simulink model "4ex4_sim"  (R2015b)
settings: Solver=VariableStepAuto  StartTime=0.0  StopTime=5  RelTol=1e-3
values from neighbouring files (symbols this model uses):
  J = (J1 + J2)    (= 3.6e-05)    [ex1.m]    (also in ex2.m; ex3.m; ex4.m)
  motor_L = motor_pars    [ex1.m]    (also in ex2.m; ex3.m; ex4.m)
  n = 5    [ex1.m]    (also in ex2.m; ex3.m; ex4.m; ex5.m)
  sim_zoh_sample_time = 0    [ex2.m]    (also in ex3.m; ex4.m = 0.001; exall.m)
libraries: simulink x1
settings Model: Creator=gabras  LastModifiedBy=Lamn
settings SolverCC: ZeroCrossAlgorithm=Adaptive
settings DataIOCC: SaveFormat=Array
settings DebuggingCC: SolverPrmCheckMsg=warning
settings HardwareCC: ProdBitPerPointer=32  ProdLargestAtomicFloat=None  ProdIntDivRoundTo=Undefined  ProdEndianess=Unspecified  ProdWordSize=32  ProdHWDeviceType=32-bit Generic
settings GRTTargetCC: GeneratePreprocessorConditionals=Disable all
settings ConfigComp: CovModelRefEnable=Off  CovSFcnEnable=off

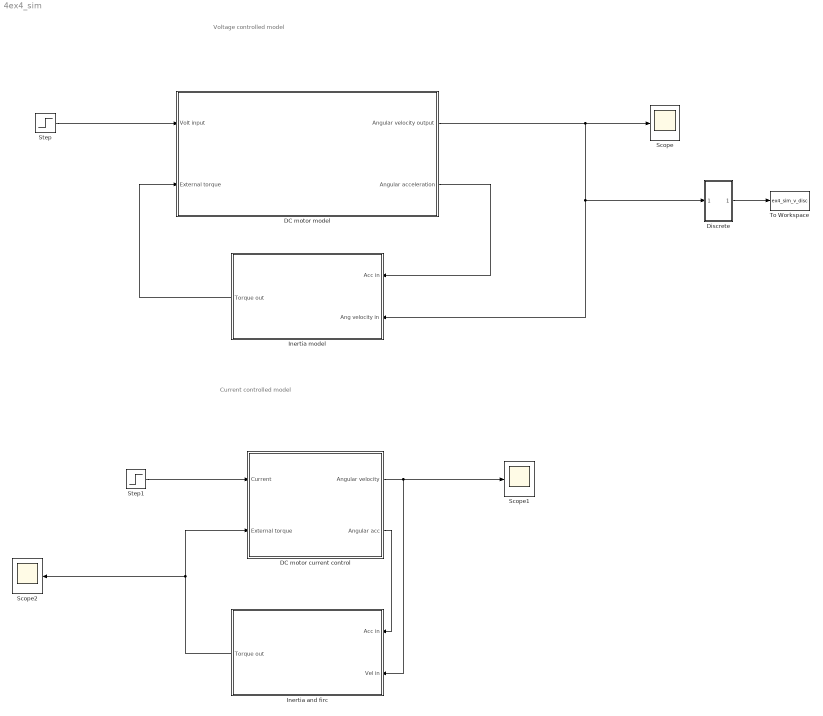
== system 4ex4_sim ==
  note: Current controlled model
  note: Voltage controlled model
  "DC motor current control " : Subsystem
  DC motor model : Subsystem
  Discrete : Subsystem
  Inertia and firc : Subsystem
  Inertia model : Subsystem
  Scope : Scope
  Scope1 : Scope
  Scope2 : Scope
  Step : Step  Time=0  SampleTime=0
  Step1 : Step  Time=0  SampleTime=0
  To Workspace : ToWorkspace  VariableName=ex4_sim_v_disc  SaveFormat=Timeseries  SampleTime=-1
  wires:
  Step/1 -> DC motor model/1("Volt input ")
  DC motor model/1("Angular velocity output ") -> Discrete/1(In1), Inertia model/2(Ang velocity in), Scope/1
  Inertia model/1(Torque out) -> DC motor model/2(External torque)
  DC motor model/2("Angular acceleration ") -> Inertia model/1(Acc in)
  Step1/1 -> "DC motor current control "/1(Current)
  "DC motor current control "/1(Angular velocity) -> Scope1/1, Inertia and firc/2(Vel in)
  "DC motor current control "/2(Angular acc) -> Inertia and firc/1(Acc in)
  Inertia and firc/1(Torque out) -> Scope2/1, "DC motor current control "/2(External torque)
  Discrete/1(Out1) -> To Workspace/1

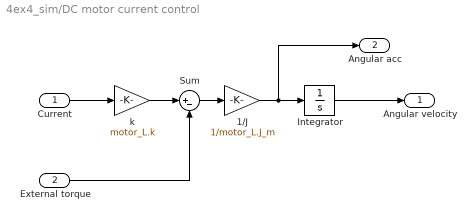
== system 4ex4_sim/DC motor current control  ==
  Current : Inport
  External torque : Inport  Port=2
  1/J : Gain  Gain=1/motor_L.J_m
  Integrator : Integrator
  Sum : Sum  Inputs=|+-
  "k " : Gain  Gain=motor_L.k
  Angular velocity : Outport
  Angular acc : Outport  Port=2
  wires:
  Current/1 -> "k "/1
  External torque/1 -> Sum/2
  "k "/1 -> Sum/1
  Sum/1 -> 1/J/1
  1/J/1 -> Angular acc/1, Integrator/1
  Integrator/1 -> Angular velocity/1

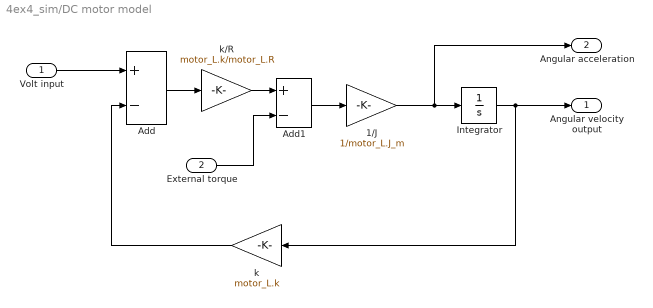
== system 4ex4_sim/DC motor model ==
  "Volt input " : Inport
  External torque : Inport  Port=2
  1/J : Gain  Gain=1/motor_L.J_m
  Add : Sum  Inputs=+-
  Add1 : Sum  Inputs=+-
  Integrator : Integrator
  k : Gain  Gain=motor_L.k
  "k/R " : Gain  Gain=motor_L.k/motor_L.R
  "Angular velocity output " : Outport
  "Angular acceleration " : Outport  Port=2
  wires:
  "Volt input "/1 -> Add/1
  k/1 -> Add/2
  Add/1 -> "k/R "/1
  "k/R "/1 -> Add1/1
  Add1/1 -> 1/J/1
  1/J/1 -> "Angular acceleration "/1, Integrator/1
  Integrator/1 -> k/1, "Angular velocity output "/1
  External torque/1 -> Add1/2

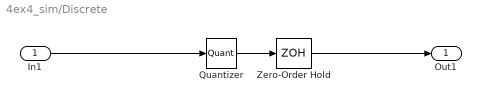
== system 4ex4_sim/Discrete ==
  In1 : Inport
  Quantizer : Quantizer  QuantizationInterval=sim_quantization_interval
  Zero-Order Hold : ZeroOrderHold  SampleTime=sim_zoh_sample_time
  Out1 : Outport
  wires:
  Quantizer/1 -> Zero-Order Hold/1
  In1/1 -> Quantizer/1
  Zero-Order Hold/1 -> Out1/1

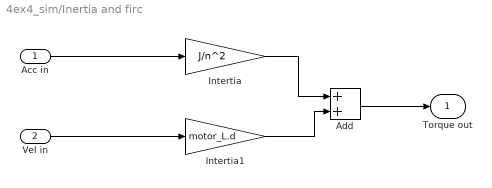
== system 4ex4_sim/Inertia and firc ==
  Acc in : Inport
  Vel in : Inport  Port=2
  Add : Sum
  Intertia : Gain  Gain=J/n^2
  Intertia1 : Gain  Gain=motor_L.d
  Torque out : Outport
  wires:
  Acc in/1 -> Intertia/1
  Vel in/1 -> Intertia1/1
  Intertia/1 -> Add/1
  Intertia1/1 -> Add/2
  Add/1 -> Torque out/1

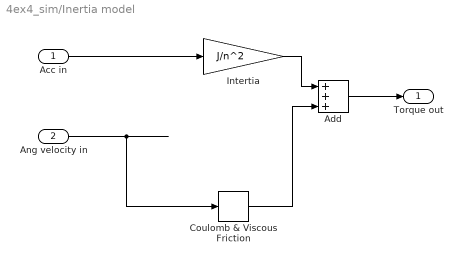
== system 4ex4_sim/Inertia model ==
  Acc in : Inport
  Ang velocity in : Inport  Port=2
  Add : Sum  Inputs=+++
  Coulomb & Viscous Friction : simulink/Discontinuities/Coulomb & Viscous Friction  offset=0.001  gain=motor_L.d
  Intertia : Gain  Gain=J/n^2
  Torque out : Outport
  wires:
  Acc in/1 -> Intertia/1
  Intertia/1 -> Add/1
  ? -> Add/2
  Ang velocity in/1 -> Coulomb & Viscous Friction/1
  Add/1 -> Torque out/1
  Coulomb & Viscous Friction/1 -> Add/3
